simulink model "Lab1_PD"  (R2019a)
settings: Solver=VariableStepAuto  StartTime=0.0  StopTime=1000  RelTol=1e-3
undefined symbols (not defined in the file or in its folder): G1, G2, Kd
settings Model: OrderedModelArguments=off  Creator=Gabe Casciano  LastModifiedBy=Gabe Casciano

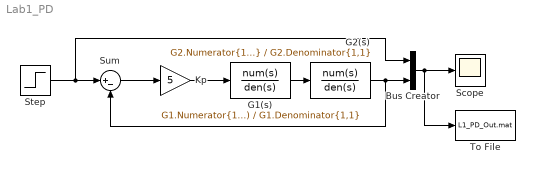
== system Lab1_PD ==
  Bus Creator : BusCreator  Inputs=2
  G1(s) : TransferFcn  Numerator=G1.Numerator{1,1}*(Kd + 1)  Denominator=G1.Denominator{1,1}
  G2(s) : TransferFcn  Numerator=G2.Numerator{1,1}  Denominator=G2.Denominator{1,1}
  Kp : Gain  Gain=5
  Scope : Scope
  Step : Step  Time=0  SampleTime=0
  Sum : Sum  Inputs=|+-
  To File : ToFile  Filename=L1_PD_Out.mat  MatrixName=L1_PD_Out  SaveFormat=Timeseries
  wires:
  Sum/1 -> Kp/1
  G1(s)/1 -> G2(s)/1
  Step/1 -> Sum/1, Bus Creator/1
  Bus Creator/1 -> To File/1, Scope/1
  G2(s)/1 -> Sum/2, Bus Creator/2
  Kp/1 -> G1(s)/1
